simulink subsystem "LuGre_Motor"  (R2022b)
settings: Solver=VariableStepAuto  StartTime=0.0  StopTime=10.0  RelTol=1e-3
model mask{motor_model=0, initial_conditions=zeros(4,1)}
  mask prompts: motor_model "Motor Parameters struct:"; initial_conditions "Motor Initial Conditions:"
settings Model: Creator=gotta  LastModifiedBy=gotta

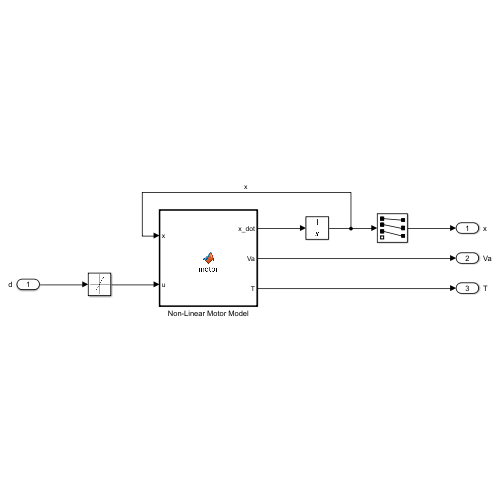
[thumbnail: Simulink's stored preview of the top-level diagram]
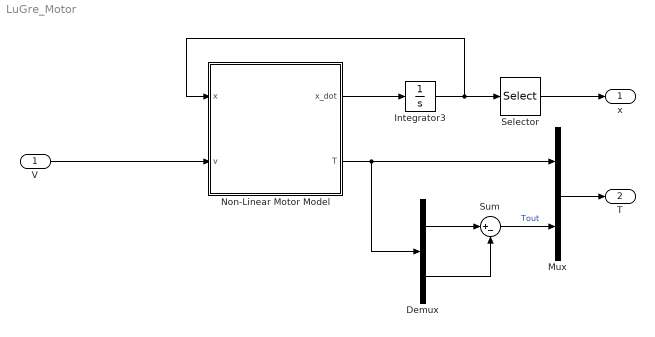
== system LuGre_Motor ==
  V : Inport
  Demux : Demux  Outputs=2
  Integrator3 : Integrator  InitialCondition=initial_conditions
  Mux : Mux  Inputs=2
  Non-Linear Motor Model : MATLAB Function  TreatAsAtomicUnit=on
  Selector : Selector  InputPortWidth=5  IndexOptions=Index vector (dialog)  Indices=[1:4]  OutputSizes=1
  Sum : Sum  Inputs=|+-
  x : Outport
  T : Outport  Port=2
  wires:
  Integrator3/1 -> Non-Linear Motor Model/1(x), Selector/1
  Non-Linear Motor Model/1(x_dot) -> Integrator3/1
  V/1 -> Non-Linear Motor Model/2(v)
  Non-Linear Motor Model/2(T) -> Mux/1, Demux/1
  Selector/1 -> x/1
  Demux/1 -> Sum/1
  Demux/2 -> Sum/2
  Sum/1 -> Mux/2  "Tout"
  Mux/1 -> T/1

== matlab function LuGre_Motor/Non-Linear Motor Model ==
  data: x input; v input; x_dot output; T output; motor_model parameter
function [x_dot, T] = motor(x, v, motor_model)

[x_dot, T] = motor_nonlinear(x, v, motor_model);
